simulink model "sampleModel2050"  (R2023a)
settings: Solver=VariableStepAuto  StartTime=0.0  StopTime=10.0  RelTol=1e-3
libraries: hdlsllib x5
settings Model: Creator=user1  LastModifiedBy=user1

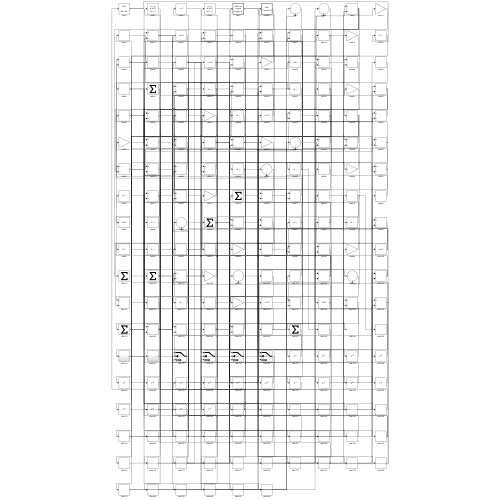
[thumbnail: Simulink's stored preview of the top-level diagram]
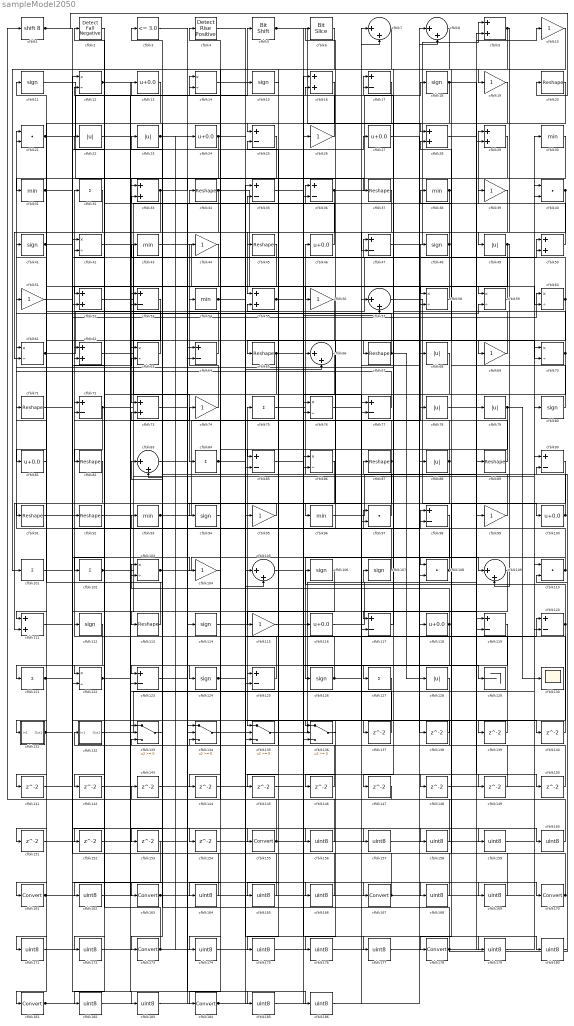
== system sampleModel2050 ==
  cfblk1 : ArithShift  BitShiftNumber=8
  cfblk{10,19,26,39,44,51,56,69,74,95,99,104,115} (13 alike) : Gain
  cfblk{13,24,27,46,81,100,116,118} (8 alike) : Bias  Bias=0.0  SaturateOnIntegerOverflow=off
  cfblk{32,75,84,101..102,121,127} (7 alike) : Sum  Inputs=+
  cfblk{12,14,42,58..61,63,70,76,86,103,122} (13 alike) : Product  Inputs=*/  RndMeth=Zero  SaturateOnIntegerOverflow=on
  cfblk{7..8,57,66,83,105,109} (7 alike) : Sum  Inputs=|++
  cfblk{11,15,18,41,48,80,94,106..107,112,114,124,126} (13 alike) : Signum
  cfblk{21,40,97,108,110} (5 alike) : DotProduct  OutDataTypeStr=Inherit: Inherit via internal rule
  cfblk{9,16,28..29,33,50,52,55,62,73,111} (11 alike) : Sum
  cfblk{20,34,37,45,65,67,71,82,87,89,91..92,113} (13 alike) : Reshape
  cfblk{17,25,35..36,47,53,64,72,77,85,90,98,117,119..120,123,125} (17 alike) : Sum  Inputs=+-
  cfblk{22..23,49,68,78..79,88,128} (8 alike) : Abs  SaturateOnIntegerOverflow=off
  cfblk129 : Terminator
  cfblk130 : Scope
  cfblk131 : Subsystem
      settings: LibrarySourceBlock=|
      | hdlsllib/Ports &
      | Subsystems/Subsystem
  cfblk132 : Subsystem
      settings: LibrarySourceBlock=|
      | hdlsllib/Ports &
      | Subsystems/Subsystem
  cfblk{133..136} (4 alike) : Switch  SaturateOnIntegerOverflow=off  InputSameDT=off
  cfblk{137..154} (18 alike) : Delay  SampleTime=1
  cfblk{155,161,163,167,170,173,178,181,184} (9 alike) : DataTypeConversion  SaturateOnIntegerOverflow=off  RndMeth=Floor
  cfblk{156..160,162,164..166,168..169,171..172,174..177,179..180,182..183,185..186} (23 alike) : DataTypeConversion  OutDataTypeStr=uint8  SaturateOnIntegerOverflow=off  RndMeth=Floor
  cfblk2 : hdlsllib/Logic and Bit Operations/Detect Fall Negative  vinit=0  OutDataTypeStr=boolean
  cfblk3 : hdlsllib/Logic and Bit Operations/Compare To Constant  relop=<=  const=3.0  OutDataTypeStr=boolean
  cfblk{30..31,38,43,54,93,96} (7 alike) : MinMax
  cfblk4 : hdlsllib/Logic and Bit Operations/Detect Rise Positive  vinit=0  OutDataTypeStr=boolean
  cfblk5 : hdlsllib/Logic and Bit Operations/Bit Shift  mode=Shift Left Logical  N=0
  cfblk6 : hdlsllib/Logic and Bit Operations/Bit Slice  lidx=7  ridx=0
  wires:
  cfblk21/1 -> cfblk13/1, cfblk104/1
  cfblk47/1 -> cfblk9/1
  cfblk38/1 -> cfblk65/1, cfblk47/2
  cfblk26/1 -> cfblk14/1
  cfblk135/1 -> cfblk107/1
  cfblk117/1 -> cfblk21/1
  cfblk67/1 -> cfblk21/2, cfblk128/1
  cfblk108/1 -> cfblk51/1, cfblk93/1
  cfblk43/1 -> cfblk59/1
  cfblk125/1 -> cfblk32/1
  cfblk83/1 -> cfblk167/1
  cfblk6/1 -> cfblk101/1
  cfblk14/1 -> cfblk5/1
  cfblk25/1 -> cfblk31/1
  cfblk57/1 -> cfblk100/1
  cfblk24/1 -> cfblk52/1, cfblk148/1, cfblk177/1
  cfblk99/1 -> cfblk87/1
  cfblk102/1 -> cfblk36/1, cfblk136/2
  cfblk37/1 -> cfblk122/1
  cfblk36/1 -> cfblk55/1, cfblk18/1
  cfblk30/1 -> cfblk173/1
  cfblk116/1 -> cfblk9/2
  cfblk88/1 -> cfblk48/1, cfblk62/1, cfblk165/1
  cfblk93/1 -> cfblk78/1, cfblk35/2
  cfblk55/1 -> cfblk77/2, cfblk179/1
  cfblk114/1 -> cfblk75/1
  cfblk72/1 -> cfblk59/2, cfblk82/1
  cfblk128/1 -> cfblk132/1(In1)
  cfblk45/1 -> cfblk111/1
  cfblk98/1 -> cfblk126/1
  cfblk106/1 -> cfblk135/1
  cfblk64/1 -> cfblk44/1
  cfblk33/1 -> cfblk102/1, cfblk37/1
  cfblk74/1 -> cfblk54/1
  cfblk29/1 -> cfblk73/1
  cfblk120/1 -> cfblk106/1, cfblk135/3
  cfblk50/1 -> cfblk29/1
  cfblk61/1 -> cfblk50/1, cfblk27/1
  cfblk90/1 -> cfblk178/1
  cfblk68/1 -> cfblk115/1
  cfblk31/1 -> cfblk136/1, cfblk53/2
  cfblk51/1 -> cfblk12/1
  cfblk63/1 -> cfblk41/1
  cfblk52/1 -> cfblk39/1
  cfblk100/1 -> cfblk46/1, cfblk72/1
  cfblk133/1 -> cfblk163/1
  cfblk17/1 -> cfblk123/1
  cfblk121/1 -> cfblk98/1, cfblk60/1, cfblk166/1
  cfblk75/1 -> cfblk66/1
  cfblk60/1 -> cfblk96/1, cfblk17/2
  cfblk10/1 -> cfblk58/1
  cfblk18/1 -> cfblk89/1, cfblk91/1
  cfblk81/1 -> cfblk11/1
  cfblk41/1 -> cfblk92/1, cfblk119/2
  cfblk13/1 -> cfblk81/1
  cfblk66/1 -> cfblk123/2
  cfblk132/1(Out1) -> cfblk80/1
  cfblk126/1 -> cfblk57/1, cfblk23/1, cfblk68/1
  cfblk9/1 -> cfblk127/1, cfblk19/1, cfblk67/1, cfblk49/1
  cfblk96/1 -> cfblk29/2
  cfblk134/1 -> cfblk120/1
  cfblk5/1 -> cfblk28/1, cfblk108/2
  cfblk95/1 -> cfblk94/1
  cfblk56/1 -> cfblk85/1
  cfblk11/1 -> cfblk95/1
  cfblk42/1 -> cfblk134/1
  cfblk46/1 -> cfblk2/1
  cfblk97/1 -> cfblk34/1
  cfblk80/1 -> cfblk28/2
  cfblk40/1 -> cfblk52/2, cfblk131/1(In1)
  cfblk104/1 -> cfblk14/2
  cfblk65/1 -> cfblk129/1, cfblk182/1
  cfblk84/1 -> cfblk66/2, cfblk149/1
  cfblk77/1 -> cfblk61/1
  cfblk3/1 -> cfblk155/1
  cfblk54/1 -> cfblk58/2, cfblk117/2, cfblk156/1
  cfblk7/1 -> cfblk184/1
  cfblk28/1 -> cfblk10/1
  cfblk109/1 -> cfblk117/1
  cfblk70/1 -> cfblk12/2, cfblk136/3
  cfblk105/1 -> cfblk170/1
  cfblk115/1 -> cfblk116/1
  cfblk62/1 -> cfblk84/1
  cfblk85/1 -> cfblk57/2
  cfblk82/1 -> cfblk111/2
  cfblk112/1 -> cfblk161/1
  cfblk86/1 -> cfblk181/1
  cfblk119/1 -> cfblk125/1
  cfblk16/1 -> cfblk25/1
  cfblk73/1 -> cfblk114/1
  cfblk110/1 -> cfblk16/2, cfblk108/1
  cfblk12/1 -> cfblk64/2, cfblk140/1
  cfblk34/1 -> cfblk122/2, cfblk118/1
  cfblk49/1 -> cfblk109/2, cfblk151/1, cfblk152/1
  cfblk59/1 -> cfblk6/1
  cfblk111/1 -> cfblk50/2
  cfblk118/1 -> cfblk103/1, cfblk153/1
  cfblk1/1 -> cfblk20/1, cfblk60/2
  cfblk103/1 -> cfblk109/1, cfblk186/1
  cfblk124/1 -> cfblk97/1, cfblk168/1
  cfblk91/1 -> cfblk113/1
  cfblk69/1 -> cfblk43/1
  cfblk87/1 -> cfblk25/2, cfblk164/1
  cfblk113/1 -> cfblk71/1
  cfblk32/1 -> cfblk61/2
  cfblk48/1 -> cfblk121/1, cfblk45/1, cfblk85/2
  cfblk131/1(Out1) -> cfblk63/2, cfblk160/1
  cfblk122/1 -> cfblk15/1, cfblk47/1, cfblk74/1
  cfblk23/1 -> cfblk69/1, cfblk70/2, cfblk97/2
  cfblk20/1 -> cfblk124/1
  cfblk79/1 -> cfblk130/1, cfblk144/1
  cfblk58/1 -> cfblk56/1
  cfblk107/1 -> cfblk33/2
  cfblk35/1 -> cfblk76/2
  cfblk92/1 -> cfblk70/1
  cfblk89/1 -> cfblk17/1
  cfblk123/1 -> cfblk137/1
  cfblk137/1 -> cfblk33/1
  cfblk27/1 -> cfblk138/1
  cfblk138/1 -> cfblk135/2
  cfblk76/1 -> cfblk139/1
  cfblk139/1 -> cfblk42/2
  cfblk140/1 -> cfblk98/2
  cfblk44/1 -> cfblk141/1
  cfblk39/1 -> cfblk142/1
  cfblk142/1 -> cfblk16/1
  cfblk144/1 -> cfblk36/2
  cfblk15/1 -> cfblk145/1
  cfblk127/1 -> cfblk146/1
  cfblk146/1 -> cfblk53/1
  cfblk19/1 -> cfblk147/1
  cfblk147/1 -> cfblk1/1
  cfblk148/1 -> cfblk110/1
  cfblk149/1 -> cfblk134/3
  cfblk78/1 -> cfblk150/1
  cfblk150/1 -> cfblk55/2
  cfblk151/1 -> cfblk134/2
  cfblk71/1 -> cfblk154/1
  cfblk154/1 -> cfblk120/2
  cfblk155/1 -> cfblk72/2, cfblk22/1
  cfblk156/1 -> cfblk3/1
  cfblk4/1 -> cfblk157/1
  cfblk157/1 -> cfblk79/1
  cfblk101/1 -> cfblk158/1
  cfblk158/1 -> cfblk4/1
  cfblk143/1 -> cfblk159/1
  cfblk159/1 -> cfblk40/1
  cfblk160/1 -> cfblk143/1
  cfblk161/1 -> cfblk40/2, cfblk63/1
  cfblk2/1 -> cfblk162/1
  cfblk162/1 -> cfblk112/1
  cfblk163/1 -> cfblk103/2, cfblk26/1
  cfblk164/1 -> cfblk133/1
  cfblk165/1 -> cfblk133/2
  cfblk166/1 -> cfblk133/3
  cfblk167/1 -> cfblk99/1, cfblk42/1
  cfblk168/1 -> cfblk83/1
  cfblk152/1 -> cfblk169/1
  cfblk169/1 -> cfblk83/2
  cfblk170/1 -> cfblk38/1, cfblk76/1
  cfblk53/1 -> cfblk171/1
  cfblk171/1 -> cfblk105/1
  cfblk153/1 -> cfblk172/1
  cfblk172/1 -> cfblk105/2
  cfblk173/1 -> cfblk62/2, cfblk125/2, cfblk24/1
  cfblk94/1 -> cfblk174/1
  cfblk174/1 -> cfblk30/1
  cfblk8/1 -> cfblk175/1
  cfblk175/1 -> cfblk119/1
  cfblk136/1 -> cfblk176/1
  cfblk176/1 -> cfblk8/1
  cfblk177/1 -> cfblk8/2
  cfblk178/1 -> cfblk110/2, cfblk73/2
  cfblk179/1 -> cfblk90/1
  cfblk145/1 -> cfblk180/1
  cfblk180/1 -> cfblk90/2
  cfblk181/1 -> cfblk64/1, cfblk88/1
  cfblk182/1 -> cfblk86/1
  cfblk141/1 -> cfblk183/1
  cfblk183/1 -> cfblk86/2
  cfblk184/1 -> cfblk35/1, cfblk77/1
  cfblk22/1 -> cfblk185/1
  cfblk185/1 -> cfblk7/1
  cfblk186/1 -> cfblk7/2

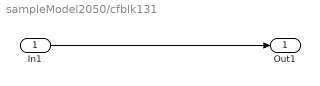
== system sampleModel2050/cfblk131 ==
  In1 : Inport
  Out1 : Outport
  wires:
  In1/1 -> Out1/1

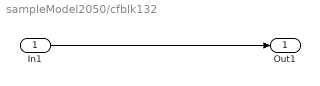
== system sampleModel2050/cfblk132 ==
  In1 : Inport
  Out1 : Outport
  wires:
  In1/1 -> Out1/1
